simulink model "sampleModel1521"  (R2023a)
settings: Solver=VariableStepAuto  StartTime=0.0  StopTime=10.0  RelTol=1e-3
libraries: hdlsllib x11, simulink x3
settings Model: Creator=user1  LastModifiedBy=user1

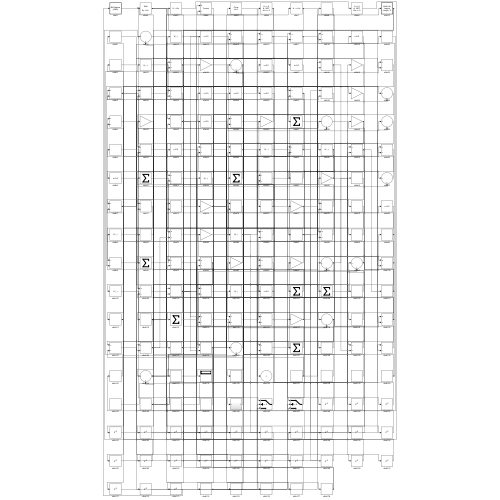
[thumbnail: Simulink's stored preview of the top-level diagram]
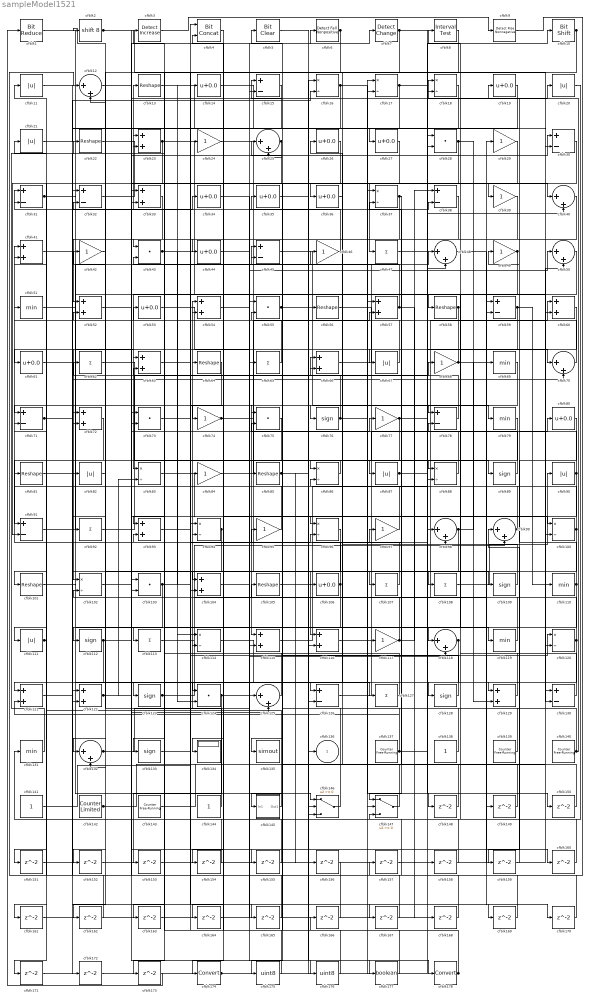
== system sampleModel1521 ==
  cfblk1 : hdlsllib/Logic and Bit Operations/Bit Reduce  mode=AND
  cfblk10 : hdlsllib/Logic and Bit Operations/Bit Shift  mode=Shift Left Logical  N=0
  cfblk{16..18,37,83,86,88,94,96,100,102,114,120} (13 alike) : Product  Inputs=*/  RndMeth=Zero  SaturateOnIntegerOverflow=on
  cfblk{13,22,56,58,64,81,85,101,105} (9 alike) : Reshape
  cfblk{28,43,55,73,75,103,124} (7 alike) : DotProduct  OutDataTypeStr=Inherit: Inherit via internal rule
  cfblk{23,33,41,52,54,57,60,63,66,72,93,104,115..116,121..122,129} (17 alike) : Sum
  cfblk{14,19,26..27,34..36,44,53,61,80,106} (12 alike) : Bias  Bias=0.0  SaturateOnIntegerOverflow=off
  cfblk{47,62,65,92,107..108,113,127} (8 alike) : Sum  Inputs=+
  cfblk{76,89,109,112,123,128,133} (7 alike) : Signum
  cfblk{11,20..21,67,82,87,90,111} (8 alike) : Abs  SaturateOnIntegerOverflow=off
  cfblk{51,69,79,110,119,131} (6 alike) : MinMax
  cfblk{24,29,39,42,46,49,68,74,77,84,95,97,117} (13 alike) : Gain
  cfblk{12,25,40,48,50,70,98..99,118,125,132} (11 alike) : Sum  Inputs=|++
  cfblk{15,30..32,38,45,59,71,78,91,126,130} (12 alike) : Sum  Inputs=+-
  cfblk134 : Display
  cfblk135 : ToWorkspace  VariableName=simout  SaveFormat=Timeseries  SampleTime=-1
  cfblk{137,139..140,143} (4 alike) : hdlsllib/Sources/Counter Free-Running  NumBits=16  tsamp=-1
  cfblk138 : Constant  SampleTime=-1
  cfblk141 : Constant  SampleTime=-1
  cfblk142 : hdlsllib/Sources/Counter Limited  uplimit=7  tsamp=-1
  cfblk144 : Constant  SampleTime=-1
  cfblk145 : Subsystem
      settings: LibrarySourceBlock=|
      | hdlsllib/Ports &
      | Subsystems/Subsystem
  cfblk146 : Switch  SaturateOnIntegerOverflow=off  InputSameDT=off
  cfblk147 : Switch  SaturateOnIntegerOverflow=off  InputSameDT=off
  cfblk{148..173} (26 alike) : Delay  SampleTime=1
  cfblk174 : DataTypeConversion  SaturateOnIntegerOverflow=off  RndMeth=Floor
  cfblk175 : DataTypeConversion  OutDataTypeStr=uint8  SaturateOnIntegerOverflow=off  RndMeth=Floor
  cfblk176 : DataTypeConversion  OutDataTypeStr=uint8  SaturateOnIntegerOverflow=off  RndMeth=Floor
  cfblk177 : DataTypeConversion  OutDataTypeStr=boolean  SaturateOnIntegerOverflow=off  RndMeth=Floor
  cfblk178 : DataTypeConversion  SaturateOnIntegerOverflow=off  RndMeth=Floor
  cfblk2 : ArithShift  BitShiftNumber=8
  cfblk3 : simulink/Logic and Bit Operations/Detect Increase  vinit=0.0  OutDataTypeStr=boolean
      settings: LibrarySourceBlock=|
      | hdlsllib/Logic and Bit
      | Operations/Detect
      | Increase
  cfblk4 : hdlsllib/Logic and Bit Operations/Bit Concat  numInputs=2
  cfblk5 : simulink/Logic and Bit Operations/Bit Clear  iBit=0
      settings: LibrarySourceBlock=|
      | hdlsllib/Logic and Bit
      | Operations/Bit Clear
  cfblk6 : hdlsllib/Logic and Bit Operations/Detect Fall Nonpositive  vinit=0  OutDataTypeStr=boolean
  cfblk7 : simulink/Logic and Bit Operations/Detect Change  vinit=0  OutDataTypeStr=boolean
      settings: LibrarySourceBlock=|
      | hdlsllib/Logic and Bit
      | Operations/Detect
      | Change
  cfblk8 : hdlsllib/Logic and Bit Operations/Interval Test  IntervalClosedRight=on  uplimit=0.5  IntervalClosedLeft=on  lowlimit=-0.5  OutDataTypeStr=boolean
  cfblk9 : hdlsllib/Logic and Bit Operations/Detect Rise Nonnegative  vinit=0  OutDataTypeStr=boolean
  cfblk136 : Outport  VectorParamsAs1DForOutWhenUnconnected=off
  wires:
  cfblk14/1 -> cfblk27/1
  cfblk23/1 -> cfblk58/1, cfblk132/1
  cfblk1/1 -> cfblk146/1
  cfblk24/1 -> cfblk86/1
  cfblk107/1 -> cfblk41/1
  cfblk108/1 -> cfblk90/1
  cfblk82/1 -> cfblk2/1
  cfblk32/1 -> cfblk36/1
  cfblk77/1 -> cfblk91/1, cfblk150/1
  cfblk91/1 -> cfblk48/1
  cfblk126/1 -> cfblk60/1
  cfblk45/1 -> cfblk78/1
  cfblk140/1 -> cfblk19/1, cfblk97/1
  cfblk72/1 -> cfblk101/1
  cfblk30/1 -> cfblk47/1
  cfblk143/1 -> cfblk56/1
  cfblk101/1 -> cfblk127/1
  cfblk92/1 -> cfblk68/1
  cfblk103/1 -> cfblk112/1, cfblk114/1, cfblk14/1, cfblk96/2, cfblk167/1
  cfblk131/1 -> cfblk22/1
  cfblk50/1 -> cfblk83/1
  cfblk46/1 -> cfblk13/1
  cfblk109/1 -> cfblk46/1
  cfblk7/1 -> cfblk126/1, cfblk70/1
  cfblk75/1 -> cfblk123/1
  cfblk132/1 -> cfblk54/1, cfblk6/1, cfblk177/1
  cfblk123/1 -> cfblk99/2, cfblk23/2
  cfblk81/1 -> cfblk113/1
  cfblk2/1 -> cfblk60/2, cfblk125/2, cfblk100/2
  cfblk120/1 -> cfblk42/1, cfblk12/2, cfblk151/1
  cfblk66/1 -> cfblk28/1
  cfblk94/1 -> cfblk132/2, cfblk163/1
  cfblk69/1 -> cfblk115/1
  cfblk127/1 -> cfblk53/1
  cfblk60/1 -> cfblk102/1
  cfblk29/1 -> cfblk91/2
  cfblk95/1 -> cfblk31/1
  cfblk25/1 -> cfblk121/1, cfblk164/1
  cfblk146/1 -> cfblk45/1
  cfblk115/1 -> cfblk48/2
  cfblk97/1 -> cfblk86/2
  cfblk90/1 -> cfblk134/1, cfblk49/1
  cfblk33/1 -> cfblk52/1
  cfblk110/1 -> cfblk18/1, cfblk54/2, cfblk173/1
  cfblk84/1 -> cfblk17/1
  cfblk116/1 -> cfblk80/1
  cfblk74/1 -> cfblk109/1, cfblk50/1, cfblk176/1
  cfblk56/1 -> cfblk88/1
  cfblk62/1 -> cfblk89/1
  cfblk20/1 -> cfblk131/1
  cfblk130/1 -> cfblk55/2
  cfblk43/1 -> cfblk130/2, cfblk124/2, cfblk169/1
  cfblk5/1 -> cfblk178/1
  cfblk144/1 -> cfblk102/2
  cfblk57/1 -> cfblk3/1, cfblk158/1
  cfblk125/1 -> cfblk94/2
  cfblk93/1 -> cfblk108/1
  cfblk47/1 -> cfblk79/1
  cfblk142/1 -> cfblk33/1, cfblk29/1, cfblk50/2
  cfblk59/1 -> cfblk147/1, cfblk110/1
  cfblk68/1 -> cfblk67/1, cfblk170/1
  cfblk147/1 -> cfblk66/1
  cfblk28/1 -> cfblk61/1, cfblk129/2
  cfblk100/1 -> cfblk64/1, cfblk145/1(In1)
  cfblk122/1 -> cfblk30/1, cfblk83/2
  cfblk86/1 -> cfblk82/1
  cfblk10/1 -> cfblk18/2, cfblk133/1
  cfblk15/1 -> cfblk74/1
  cfblk124/1 -> cfblk118/2, cfblk38/2, cfblk153/1
  cfblk16/1 -> cfblk43/1, cfblk148/1
  cfblk141/1 -> cfblk24/1
  cfblk17/1 -> cfblk92/1, cfblk100/1
  cfblk98/1 -> cfblk116/1, cfblk69/1
  cfblk87/1 -> cfblk10/1, cfblk168/1
  cfblk133/1 -> cfblk120/1
  cfblk65/1 -> cfblk51/1
  cfblk104/1 -> cfblk125/1
  cfblk117/1 -> cfblk35/1, cfblk38/1
  cfblk112/1 -> cfblk77/1, cfblk20/1, cfblk119/1, cfblk161/1
  cfblk99/1 -> cfblk81/1, cfblk129/1
  cfblk83/1 -> cfblk136/1
  cfblk6/1 -> cfblk72/1, cfblk93/1
  cfblk19/1 -> cfblk33/2
  cfblk85/1 -> cfblk57/2, cfblk156/1
  cfblk52/1 -> cfblk7/1
  cfblk54/1 -> cfblk88/2
  cfblk51/1 -> cfblk63/1
  cfblk138/1 -> cfblk62/1
  cfblk89/1 -> cfblk8/1
  cfblk145/1(Out1) -> cfblk41/2
  cfblk111/1 -> cfblk11/1, cfblk171/1
  cfblk76/1 -> cfblk57/1, cfblk43/2
  cfblk40/1 -> cfblk104/1
  cfblk4/1 -> cfblk174/1
  cfblk70/1 -> cfblk26/1
  cfblk128/1 -> cfblk95/1
  cfblk55/1 -> cfblk87/1, cfblk25/2
  cfblk114/1 -> cfblk126/2
  cfblk26/1 -> cfblk72/2
  cfblk106/1 -> cfblk52/2, cfblk116/2
  cfblk49/1 -> cfblk135/1, cfblk118/1
  cfblk137/1 -> cfblk98/2, cfblk114/2, cfblk121/2
  cfblk39/1 -> cfblk124/1
  cfblk61/1 -> cfblk23/1
  cfblk31/1 -> cfblk115/2, cfblk106/1
  cfblk78/1 -> cfblk15/1
  cfblk35/1 -> cfblk40/1
  cfblk38/1 -> cfblk44/1
  cfblk22/1 -> cfblk120/2
  cfblk63/1 -> cfblk84/1
  cfblk88/1 -> cfblk25/1
  cfblk129/1 -> cfblk105/1
  cfblk21/1 -> cfblk16/2
  cfblk64/1 -> cfblk111/1
  cfblk118/1 -> cfblk128/1, cfblk154/1
  cfblk113/1 -> cfblk59/2
  cfblk12/1 -> cfblk39/1
  cfblk34/1 -> cfblk65/1
  cfblk13/1 -> cfblk37/1
  cfblk36/1 -> cfblk96/1
  cfblk18/1 -> cfblk122/2
  cfblk37/1 -> cfblk73/2, cfblk107/1
  cfblk53/1 -> cfblk85/1
  cfblk67/1 -> cfblk21/1
  cfblk105/1 -> cfblk40/2
  cfblk119/1 -> cfblk32/2
  cfblk79/1 -> cfblk103/2
  cfblk58/1 -> cfblk71/1, cfblk76/1
  cfblk8/1 -> cfblk104/2
  cfblk3/1 -> cfblk9/1
  cfblk71/1 -> cfblk34/1, cfblk70/2
  cfblk73/1 -> cfblk75/1
  cfblk139/1 -> cfblk31/2
  cfblk11/1 -> cfblk30/2
  cfblk148/1 -> cfblk66/2
  cfblk48/1 -> cfblk149/1
  cfblk149/1 -> cfblk45/2
  cfblk150/1 -> cfblk37/2
  cfblk151/1 -> cfblk55/1
  cfblk42/1 -> cfblk152/1
  cfblk152/1 -> cfblk59/1
  cfblk153/1 -> cfblk16/1
  cfblk154/1 -> cfblk122/1
  cfblk102/1 -> cfblk155/1
  cfblk155/1 -> cfblk103/1
  cfblk156/1 -> cfblk12/1
  cfblk9/1 -> cfblk157/1
  cfblk157/1 -> cfblk130/1
  cfblk158/1 -> cfblk75/2
  cfblk80/1 -> cfblk159/1
  cfblk159/1 -> cfblk99/1
  cfblk44/1 -> cfblk160/1
  cfblk160/1 -> cfblk78/2
  cfblk161/1 -> cfblk15/2
  cfblk96/1 -> cfblk162/1
  cfblk162/1 -> cfblk32/1
  cfblk163/1 -> cfblk28/2
  cfblk164/1 -> cfblk146/2
  cfblk121/1 -> cfblk165/1
  cfblk165/1 -> cfblk94/1
  cfblk166/1 -> cfblk73/1
  cfblk167/1 -> cfblk71/2
  cfblk168/1 -> cfblk147/2
  cfblk169/1 -> cfblk63/2
  cfblk170/1 -> cfblk147/3
  cfblk171/1 -> cfblk146/3
  cfblk41/1 -> cfblk172/1
  cfblk172/1 -> cfblk17/2
  cfblk173/1 -> cfblk1/1
  cfblk174/1 -> cfblk117/1, cfblk98/1
  cfblk27/1 -> cfblk175/1
  cfblk175/1 -> cfblk4/1
  cfblk176/1 -> cfblk4/2
  cfblk177/1 -> cfblk5/1
  cfblk178/1 -> cfblk166/1, cfblk93/2

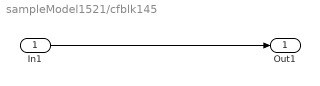
== system sampleModel1521/cfblk145 ==
  In1 : Inport
  Out1 : Outport
  wires:
  In1/1 -> Out1/1
